simulink library "util_clock_lib"  (R2014b)
settings: Solver=ode45  SolverMode=SingleTasking  StartTime=0.0  StopTime=10.0  RelTol=1e-3
undefined symbols (not defined in the file): tim_initial_met_second, tim_simulation_sample_time
libraries: util_clock_lib x2
settings Model: Creator=dviazzo  LastModifiedBy=mstewart

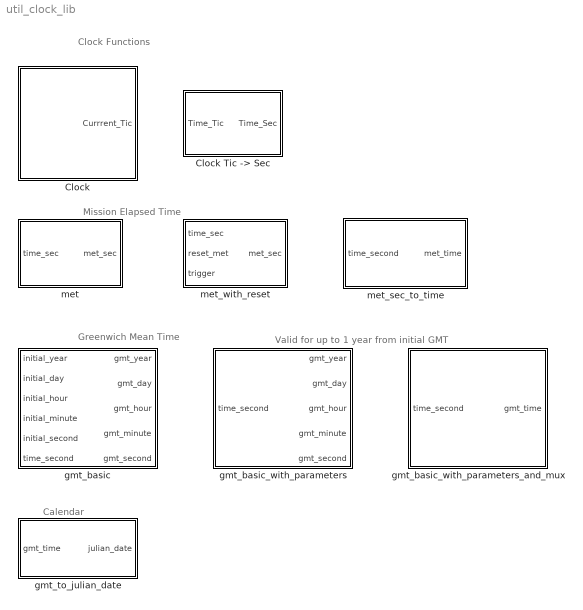
== system util_clock_lib ==
  note: Clock Functions
  note: Mission Elapsed Time
  note: Greenwich Mean Time
  note: Valid for up to 1 year from initial GMT
  note: Calendar
  Clock : Subsystem  mask{Clock_Sample_Time=tim_simulation_sample_time}
      mask prompts: Clock_Sample_Time "Enter Clock Increment Time Period"
      mask init:
      | if isempty(Clock_Sample_Time)
      |    Clock_Sample_Time = 1;
      | end
      mask Display:
      | plot(0.5+.25*sin([0:.2:(2*pi+.2)]),0.5+.25*cos([0:.2:(2*pi+.2)]));
      | plot([.5,.5],[.5,.7])
      | plot([.5,.7],[.5,.5])
      | plot([.75,.75],[.75,.95])
      | plot([.75,.95],[.75,.75])
      | plot([.75,.78,.78,.81,.81,.84,.84,.87,.87,.90,.90,.93,.93],[.75,.75,.78,.78,.81,.81,.84,.84,.87,.87,.90,.90,.93])
      | port_label('output',1,'Tic')
      | text(.05,.98,sprintf('%.0f Hz', 1/Clock_Sample_Time),...
      |     'HorizontalAlignment','Left',...
      | 	'VerticalAlignment','top')
      | text(.98,.02,sprintf('Ts = %.4f s', Clock_Sample_Time),...
      |     'HorizontalAlignment','Right',...
      | 	'VerticalAlignment','bottom')
      | color('blue')
      | text(0.05,0.02,'NASA',...
      |  	'HorizontalAlignment','Left',...
      | 	'VerticalAlignment','bottom')
  "Clock Tic -> Sec" : Subsystem  mask{Clock_Sample_Time=tim_simulation_sample_time}
      mask prompts: Clock_Sample_Time "Enter Clock Increment Time Period"
      mask init:
      | if isempty(Clock_Sample_Time)
      |    Clock_Sample_Time = 1;
      | end
      mask Display:
      | disp(sprintf('1 tic = %.4f s',Clock_Sample_Time))
      | color('blue')
      | text(0.05,0.02,'NASA',...
      |  	'HorizontalAlignment','Left',...
      | 	'VerticalAlignment','bottom')
  gmt_basic : Subsystem
      mask Display:
      | color('blue')
      | text(0.5,0.98,'NASA',...
      |  	'HorizontalAlignment','center',...
      | 	'VerticalAlignment','top')
  gmt_basic_with_parameters : Subsystem  mask{i_year=2007, i_day=1, i_hour=0, i_minute=0, i_second=0}
      mask prompts: i_year "Enter initial GMT year"; i_day "Enter initial GMT day"; i_hour "Enter initial GMT hour"; i_minute "Enter initial GMT minute"; i_second "Enter initial GMT second"
      mask help:
      | Greenwich Mean Time (GMT)
      | Valid for up to 1 year after initial date assuming that the initial date is in the GMT format (i.e. i_second <60, etc.)
      mask init:
      | if isempty(i_year) | (i_year == 0)
      |    i_year = 2007;
      | end
      | if isempty(i_day) | (i_day == 0)
      |    i_day = 1;
      | end
      | if isempty(i_hour)
      |    i_hour = 0;
      | end
      | if isempty(i_minute)
      |    i_minute = 0;
      | end
      | if isempty(i_second)
      |    i_second = 0;
      | end
      mask Display:
      | color('blue')
      | text(0.05,0.02,'NASA',...
      |  	'HorizontalAlignment','Left',...
      | 	'VerticalAlignment','bottom')
  gmt_basic_with_parameters_and_mux : Subsystem  mask{i_year=2007, i_day=1, i_hour=0, i_minute=0, i_second=0}
      mask prompts: i_year "Enter initial GMT year"; i_day "Enter initial GMT day"; i_hour "Enter initial GMT hour"; i_minute "Enter initial GMT minute"; i_second "Enter initial GMT second"
      mask help:
      | Greenwich Mean Time (GMT)
      | Valid for up to 1 year after initial date assuming that the initial date is in the GMT format (i.e. i_second <60, etc.)
      mask init: same as util_clock_lib/gmt_basic_with_parameters
      mask Display:
      | color('blue')
      | text(0.05,0.02,'NASA',...
      |  	'HorizontalAlignment','Left',...
      | 	'VerticalAlignment','bottom')
  gmt_to_julian_date : Subsystem
      mask Display:
      | color('blue')
      | text(0.05,0.02,'NASA',...
      |  	'HorizontalAlignment','Left',...
      | 	'VerticalAlignment','bottom')
  met : Subsystem  mask{initial_met=0}
      mask prompts: initial_met "Initial Mission Elapsed Time (sec)"
      mask init:
      | if isempty(Initial_MET)
      |    Initial_MET = 0;
      | end
      mask Display:
      | color('blue')
      | text(0.05,0.02,'NASA',...
      |  	'HorizontalAlignment','Left',...
      | 	'VerticalAlignment','bottom')
  met_sec_to_time : Subsystem
      mask Display:
      | color('blue')
      | text(0.05,0.02,'NASA',...
      |  	'HorizontalAlignment','Left',...
      | 	'VerticalAlignment','bottom')
  met_with_reset : Subsystem  mask{initial_met=tim_initial_met_second}
      mask prompts: initial_met "Initial Mission Elapsed Time (sec)"
      mask init:
      | if isempty(initial_met)
      |    initial_met = 0;
      | end
      mask Display:
      | color('blue')
      | text(0.95,0.02,'NASA',...
      |  	'HorizontalAlignment','right',...
      | 	'VerticalAlignment','bottom')

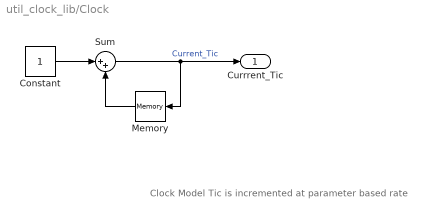
== system util_clock_lib/Clock ==
  note: Clock Model
      | Tic is incremented at parameter based rate
  Constant : Constant
  Memory : Memory  X0=-1  InheritSampleTime=on  StateIdentifier=Previous_Tic
      settings: RTWStateStorageClass=ImportedExtern
  Sum : Sum  Inputs=|++  SampleTime=Clock_Sample_Time
  Currrent_Tic : Outport  PortDimensions=1
  wires:
  Memory/1 -> Sum/2
  Sum/1 -> Memory/1, Currrent_Tic/1  "Current_Tic"
  Constant/1 -> Sum/1

== system util_clock_lib/Clock Tic -> Sec ==
  Time_Tic : Inport
  Constant : Constant  Value=Clock_Sample_Time
  Product : Product  RndMeth=Zero
  Time_Sec : Outport
  wires:
  Constant/1 -> Product/2
  Time_Tic/1 -> Product/1  "Time_Tic"
  Product/1 -> Time_Sec/1

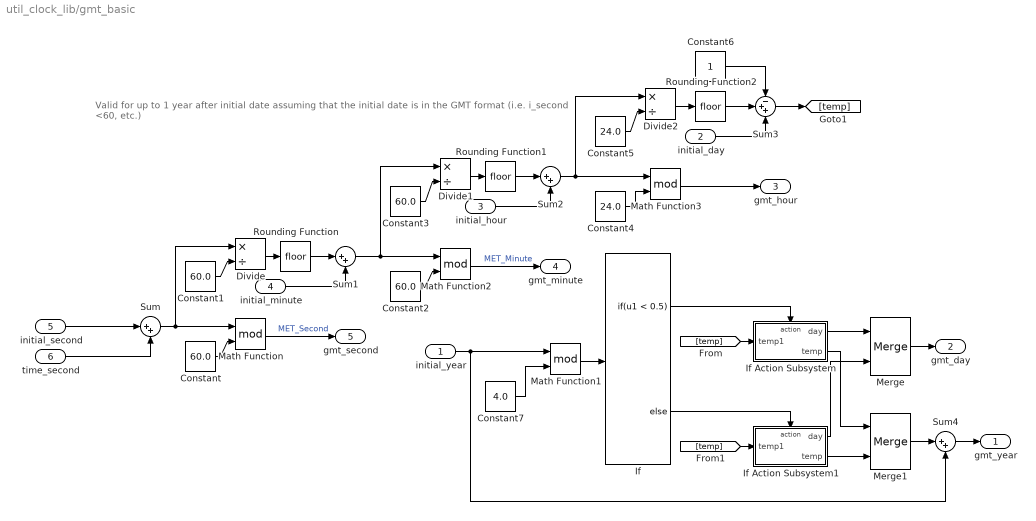
== system util_clock_lib/gmt_basic ==
  note: Valid for up to 1 year after initial date
      | assuming that the initial date is in the GMT format (i.e. i_second <60, etc.)
  initial_year : Inport
  initial_day : Inport  Port=2
  initial_hour : Inport  Port=3
  initial_minute : Inport  Port=4
  initial_second : Inport  Port=5
  time_second : Inport  Port=6
  Constant{,1..3} (4 alike) : Constant  Value=60.0
  Constant4 : Constant  Value=24.0
  Constant5 : Constant  Value=24.0
  Constant6 : Constant
  Constant7 : Constant  Value=4.0
  Divide : Product  Inputs=*/
  Divide1 : Product  Inputs=*/
  Divide2 : Product  Inputs=*/
  If : If  IfExpression=u1 < 0.5
  If Action Subsystem : Subsystem  TreatAsAtomicUnit=on
  If Action Subsystem1 : Subsystem  TreatAsAtomicUnit=on
  Math Function{,1..3} (4 alike) : Math  Operator=mod  SaturateOnIntegerOverflow=on
  Merge : Merge
  Merge1 : Merge
  Rounding Function : Rounding
  Rounding Function1 : Rounding
  Rounding Function2 : Rounding
  Sum{,1..2,4} (4 alike) : Sum  Inputs=|++
  Sum3 : Sum  Inputs=-++
  gmt_year : Outport
  gmt_day : Outport  Port=2
  gmt_hour : Outport  Port=3
  gmt_minute : Outport  Port=4
  gmt_second : Outport  Port=5
  wires:
  Sum4/1 -> gmt_year/1
  Merge1/1 -> Sum4/1
  Merge/1 -> gmt_day/1
  If Action Subsystem1/2(temp) -> Merge1/2
  If Action Subsystem/2(temp) -> Merge1/1
  If Action Subsystem1/1(day) -> Merge/2
  If Action Subsystem/1(day) -> Merge/1
  If/2 -> If Action Subsystem1/Action
  [temp] -> If Action Subsystem1/1(temp1)
  [temp] -> If Action Subsystem/1(temp1)
  Sum3/1 -> [temp]
  If/1 -> If Action Subsystem/Action
  initial_year/1 -> Sum4/2, Math Function1/1
  Math Function1/1 -> If/1
  Constant7/1 -> Math Function1/2
  Constant6/1 -> Sum3/1
  initial_day/1 -> Sum3/3
  Rounding Function2/1 -> Sum3/2
  Math Function3/1 -> gmt_hour/1
  Sum2/1 -> Divide2/1, Math Function3/1
  Divide2/1 -> Rounding Function2/1
  Constant5/1 -> Divide2/2
  Constant4/1 -> Math Function3/2
  Rounding Function1/1 -> Sum2/1
  Divide1/1 -> Rounding Function1/1
  Constant3/1 -> Divide1/2
  Sum1/1 -> Divide1/1, Math Function2/1
  Constant2/1 -> Math Function2/2
  Rounding Function/1 -> Sum1/1
  Divide/1 -> Rounding Function/1
  Constant1/1 -> Divide/2
  Constant/1 -> Math Function/2
  Sum/1 -> Divide/1, Math Function/1
  time_second/1 -> Sum/2
  initial_hour/1 -> Sum2/2
  initial_minute/1 -> Sum1/2
  initial_second/1 -> Sum/1
  Math Function2/1 -> gmt_minute/1  "MET_Minute"
  Math Function/1 -> gmt_second/1  "MET_Second"

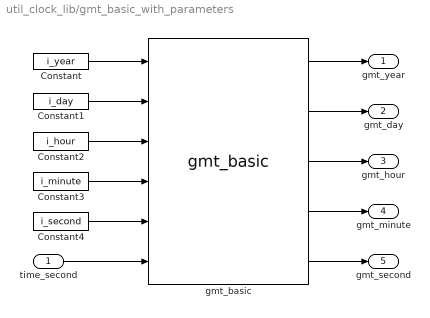
== system util_clock_lib/gmt_basic_with_parameters ==
  time_second : Inport
  Constant : Constant  Value=i_year
  Constant1 : Constant  Value=i_day
  Constant2 : Constant  Value=i_hour
  Constant3 : Constant  Value=i_minute
  Constant4 : Constant  Value=i_second
  gmt_basic : util_clock_lib/gmt_basic  SystemSampleTime=-1
  gmt_year : Outport
  gmt_day : Outport  Port=2
  gmt_hour : Outport  Port=3
  gmt_minute : Outport  Port=4
  gmt_second : Outport  Port=5
  wires:
  Constant/1 -> gmt_basic/1
  Constant1/1 -> gmt_basic/2
  Constant2/1 -> gmt_basic/3
  Constant4/1 -> gmt_basic/5
  Constant3/1 -> gmt_basic/4
  gmt_basic/5 -> gmt_second/1
  gmt_basic/4 -> gmt_minute/1
  gmt_basic/3 -> gmt_hour/1
  gmt_basic/2 -> gmt_day/1
  gmt_basic/1 -> gmt_year/1
  time_second/1 -> gmt_basic/6

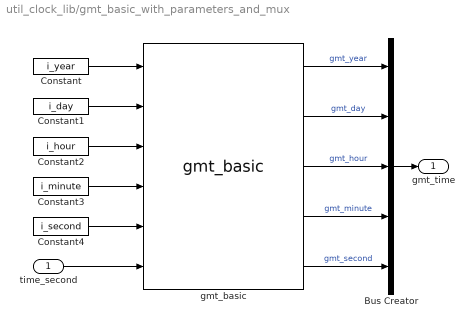
== system util_clock_lib/gmt_basic_with_parameters_and_mux ==
  time_second : Inport
  Bus Creator : BusCreator  Inputs=5
  Constant : Constant  Value=i_year
  Constant1 : Constant  Value=i_day
  Constant2 : Constant  Value=i_hour
  Constant3 : Constant  Value=i_minute
  Constant4 : Constant  Value=i_second
  gmt_basic : util_clock_lib/gmt_basic  SystemSampleTime=-1
  gmt_time : Outport
  wires:
  Bus Creator/1 -> gmt_time/1
  time_second/1 -> gmt_basic/6
  gmt_basic/1 -> Bus Creator/1  "gmt_year"
  gmt_basic/2 -> Bus Creator/2  "gmt_day"
  gmt_basic/3 -> Bus Creator/3  "gmt_hour"
  gmt_basic/4 -> Bus Creator/4  "gmt_minute"
  gmt_basic/5 -> Bus Creator/5  "gmt_second"
  Constant3/1 -> gmt_basic/4
  Constant4/1 -> gmt_basic/5
  Constant2/1 -> gmt_basic/3
  Constant1/1 -> gmt_basic/2
  Constant/1 -> gmt_basic/1

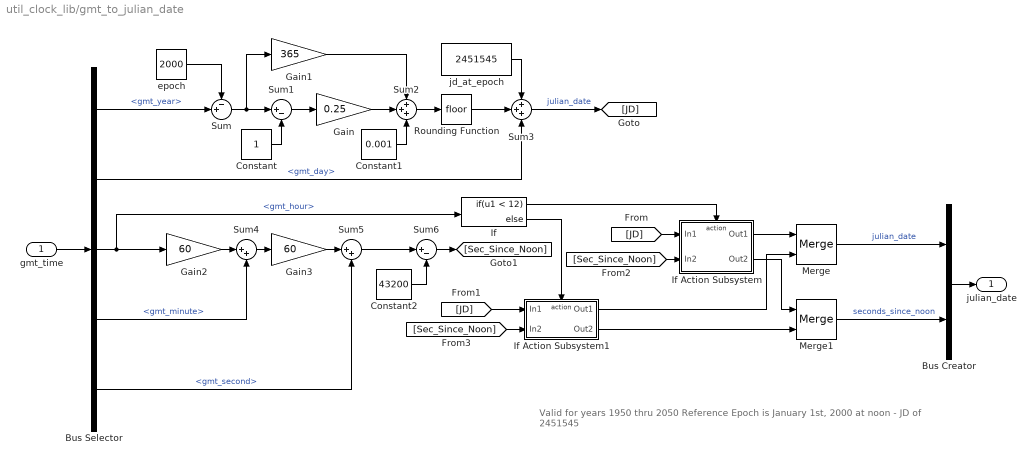
== system util_clock_lib/gmt_to_julian_date ==
  note: Valid for years 1950 thru 2050
      | Reference Epoch is January 1st, 2000 at noon - JD of 2451545
  gmt_time : Inport
  Bus Creator : BusCreator  Inputs=2
  Bus Selector : BusSelector  OutputSignals=gmt_year,gmt_day,gmt_hour,gmt_minute,gmt_second
  Constant : Constant
  Constant1 : Constant  Value=0.001
  Constant2 : Constant  Value=43200
  Gain : Gain  Gain=0.25
  Gain1 : Gain  Gain=365
  Gain2 : Gain  Gain=60
  Gain3 : Gain  Gain=60
  If : If  IfExpression=u1 < 12
  If Action Subsystem : Subsystem  TreatAsAtomicUnit=on
  If Action Subsystem1 : Subsystem  TreatAsAtomicUnit=on
  Merge : Merge
  Merge1 : Merge
  Rounding Function : Rounding
  Sum : Sum  Inputs=-+|
  Sum1 : Sum  Inputs=|+-
  Sum2 : Sum  Inputs=+++
  Sum3 : Sum  Inputs=+++
  Sum4 : Sum  Inputs=|++
  Sum5 : Sum  Inputs=|++
  Sum6 : Sum  Inputs=|+-
  epoch : Constant  Value=2000
  jd_at_epoch : Constant  Value=2451545
  julian_date : Outport
  wires:
  [Sec_Since_Noon] -> If Action Subsystem1/2(In2)
  [Sec_Since_Noon] -> If Action Subsystem/2(In2)
  [JD] -> If Action Subsystem1/1(In1)
  [JD] -> If Action Subsystem/1(In1)
  Sum6/1 -> [Sec_Since_Noon]
  Sum3/1 -> [JD]  "julian_date"
  Merge/1 -> Bus Creator/1  "julian_date"
  If/2 -> If Action Subsystem1/Action
  If/1 -> If Action Subsystem/Action
  If Action Subsystem1/2(Out2) -> Merge1/2
  If Action Subsystem/2(Out2) -> Merge1/1
  If Action Subsystem1/1(Out1) -> Merge/2
  If Action Subsystem/1(Out1) -> Merge/1
  Bus Selector/3 -> If/1, Gain2/1  "<gmt_hour>"
  Bus Selector/4 -> Sum4/2  "<gmt_minute>"
  Bus Selector/1 -> Sum/2  "<gmt_year>"
  Constant2/1 -> Sum6/2
  Sum5/1 -> Sum6/1
  Gain3/1 -> Sum5/1
  Sum4/1 -> Gain3/1
  Gain2/1 -> Sum4/1
  Rounding Function/1 -> Sum3/2
  jd_at_epoch/1 -> Sum3/1
  Sum2/1 -> Rounding Function/1
  Constant1/1 -> Sum2/3
  Gain/1 -> Sum2/2
  Gain1/1 -> Sum2/1
  Sum1/1 -> Gain/1
  Constant/1 -> Sum1/2
  Sum/1 -> Gain1/1, Sum1/1
  epoch/1 -> Sum/1
  Bus Selector/2 -> Sum3/3  "<gmt_day>"
  Bus Selector/5 -> Sum5/2  "<gmt_second>"
  Merge1/1 -> Bus Creator/2  "seconds_since_noon"
  Bus Creator/1 -> julian_date/1
  gmt_time/1 -> Bus Selector/1

== system util_clock_lib/met ==
  time_sec : Inport
  Constant : Constant  Value=initial_met
  Sum : Sum
  met_sec : Outport
  wires:
  time_sec/1 -> Sum/1
  Constant/1 -> Sum/2
  Sum/1 -> met_sec/1

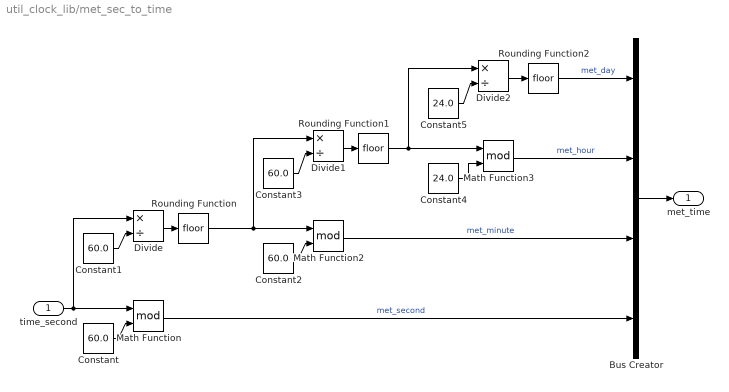
== system util_clock_lib/met_sec_to_time ==
  time_second : Inport
  Bus Creator : BusCreator
  Constant{,1..3} (4 alike) : Constant  Value=60.0
  Constant4 : Constant  Value=24.0
  Constant5 : Constant  Value=24.0
  Divide : Product  Inputs=*/
  Divide1 : Product  Inputs=*/
  Divide2 : Product  Inputs=*/
  Math Function : Math  Operator=mod  SaturateOnIntegerOverflow=on
  Math Function2 : Math  Operator=mod  SaturateOnIntegerOverflow=on
  Math Function3 : Math  Operator=mod  SaturateOnIntegerOverflow=on
  Rounding Function : Rounding
  Rounding Function1 : Rounding
  Rounding Function2 : Rounding
  met_time : Outport
  wires:
  Divide2/1 -> Rounding Function2/1
  Constant5/1 -> Divide2/2
  Rounding Function1/1 -> Divide2/1, Math Function3/1
  Constant4/1 -> Math Function3/2
  Divide1/1 -> Rounding Function1/1
  Constant3/1 -> Divide1/2
  Rounding Function/1 -> Divide1/1, Math Function2/1
  Constant2/1 -> Math Function2/2
  Divide/1 -> Rounding Function/1
  Constant1/1 -> Divide/2
  Constant/1 -> Math Function/2
  Math Function/1 -> Bus Creator/4  "met_second"
  Math Function2/1 -> Bus Creator/3  "met_minute"
  Math Function3/1 -> Bus Creator/2  "met_hour"
  Rounding Function2/1 -> Bus Creator/1  "met_day"
  time_second/1 -> Divide/1, Math Function/1
  Bus Creator/1 -> met_time/1

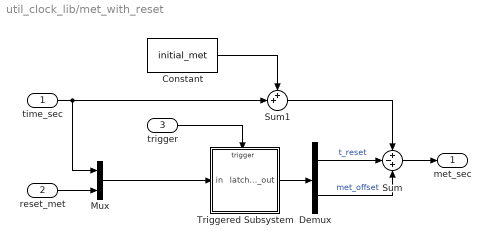
== system util_clock_lib/met_with_reset ==
  time_sec : Inport
  reset_met : Inport  Port=2
  trigger : Inport  Port=3
  Constant : Constant  Value=initial_met
  Demux : Demux  Outputs=2
  Mux : Mux  Inputs=2
  Sum : Sum  Inputs=+-+
  Sum1 : Sum  Inputs=++|
  Triggered Subsystem : Subsystem  TreatAsAtomicUnit=on
  met_sec : Outport
  wires:
  Sum/1 -> met_sec/1
  time_sec/1 -> Mux/1, Sum1/2
  Triggered Subsystem/1(latched_out) -> Demux/1
  reset_met/1 -> Mux/2
  Mux/1 -> Triggered Subsystem/1(in)
  Demux/1 -> Sum/2  "t_reset"
  Demux/2 -> Sum/3  "met_offset"
  trigger/1 -> Triggered Subsystem/Trigger
  Sum1/1 -> Sum/1
  Constant/1 -> Sum1/1

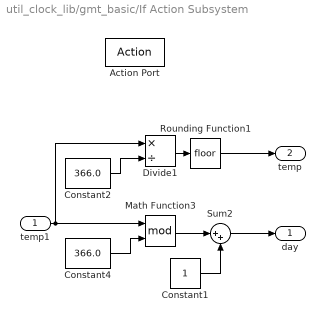
== system util_clock_lib/gmt_basic/If Action Subsystem ==
  temp1 : Inport
  Action Port : ActionPort
  Constant1 : Constant
  Constant2 : Constant  Value=366.0
  Constant4 : Constant  Value=366.0
  Divide1 : Product  Inputs=*/
  Math Function3 : Math  Operator=mod  SaturateOnIntegerOverflow=on
  Rounding Function1 : Rounding
  Sum2 : Sum  Inputs=|++
  day : Outport
  temp : Outport  Port=2
  wires:
  Rounding Function1/1 -> temp/1
  Constant2/1 -> Divide1/2
  Divide1/1 -> Rounding Function1/1
  Sum2/1 -> day/1
  Constant1/1 -> Sum2/2
  Math Function3/1 -> Sum2/1
  temp1/1 -> Divide1/1, Math Function3/1
  Constant4/1 -> Math Function3/2

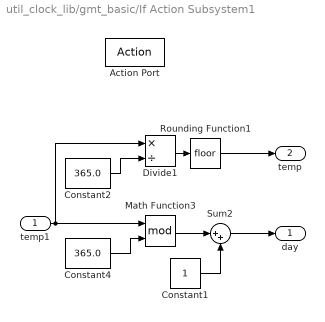
== system util_clock_lib/gmt_basic/If Action Subsystem1 ==
  temp1 : Inport
  Action Port : ActionPort
  Constant1 : Constant
  Constant2 : Constant  Value=365.0
  Constant4 : Constant  Value=365.0
  Divide1 : Product  Inputs=*/
  Math Function3 : Math  Operator=mod  SaturateOnIntegerOverflow=on
  Rounding Function1 : Rounding
  Sum2 : Sum  Inputs=|++
  day : Outport
  temp : Outport  Port=2
  wires:
  Constant4/1 -> Math Function3/2
  temp1/1 -> Math Function3/1, Divide1/1
  Math Function3/1 -> Sum2/1
  Constant1/1 -> Sum2/2
  Sum2/1 -> day/1
  Divide1/1 -> Rounding Function1/1
  Constant2/1 -> Divide1/2
  Rounding Function1/1 -> temp/1

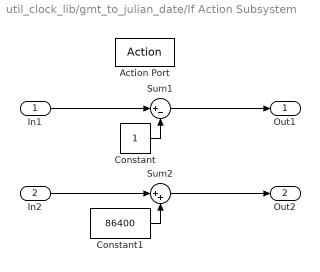
== system util_clock_lib/gmt_to_julian_date/If Action Subsystem ==
  In1 : Inport
  In2 : Inport  Port=2
  Action Port : ActionPort
  Constant : Constant
  Constant1 : Constant  Value=86400
  Sum1 : Sum  Inputs=|+-
  Sum2 : Sum  Inputs=|++
  Out1 : Outport
  Out2 : Outport  Port=2
  wires:
  Sum2/1 -> Out2/1
  In2/1 -> Sum2/1
  Constant1/1 -> Sum2/2
  Sum1/1 -> Out1/1
  In1/1 -> Sum1/1
  Constant/1 -> Sum1/2

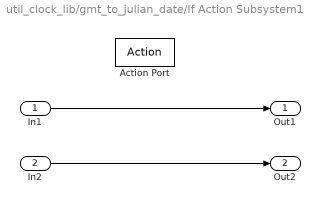
== system util_clock_lib/gmt_to_julian_date/If Action Subsystem1 ==
  In1 : Inport
  In2 : Inport  Port=2
  Action Port : ActionPort
  Out1 : Outport
  Out2 : Outport  Port=2
  wires:
  In2/1 -> Out2/1
  In1/1 -> Out1/1

== system util_clock_lib/met_with_reset/Triggered Subsystem ==
  in : Inport
  Trigger : TriggerPort
  latched_out : Outport
  wires:
  in/1 -> latched_out/1
